simulink model "spring_mass_damper"  (R2022b)
settings: Solver=VariableStepAuto  StartTime=0.0  StopTime=10.0  RelTol=1e-3
settings Model: Creator=simay  LastModifiedBy=simay

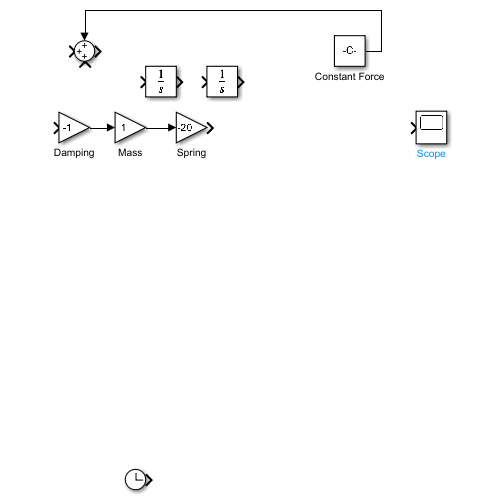
[thumbnail: Simulink's stored preview of the top-level diagram]
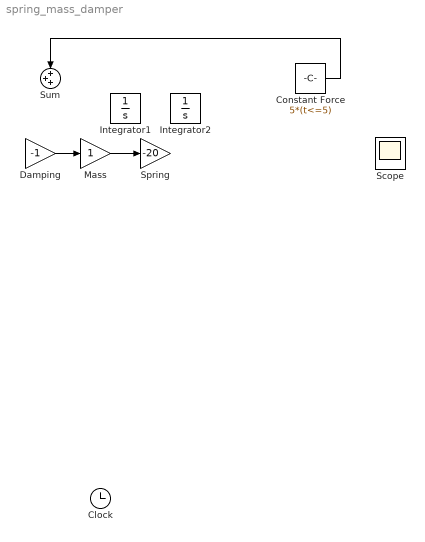
== system spring_mass_damper ==
  Clock : Clock
  Constant Force : Constant  Value=5*(t<=5)
  Damping : Gain  Gain=-1
  Integrator1 : Integrator
  Integrator2 : Integrator
  Mass : Gain
  Scope : Scope
  Spring : Gain  Gain=-20
  Sum : Sum  Inputs=+++
  wires:
  Constant Force/1 -> Sum/1
  Damping/1 -> Mass/1
  Mass/1 -> Spring/1
